simulink model "Detailed_PMSG_one_machine"  (Simulink 8.6)
settings: Solver=VariableStepAuto  StartTime=0.0  StopTime=30  FixedStep=Ts  MaxStep=Ts  RelTol=1e-3
PreLoadFcn:
  | Ts=5e-6;
InitFcn:
  | Ts=5e-6;
values from neighbouring files (symbols this model uses):
  A = c1*((c2/li-c3*u-c4)*exp(-c5/li))+c6*i    [Cpmax.m]    (also in deloaded_operation_with_pitch_angle.m = powercoefficient(tipmax,u))
undefined symbols (not defined in the file or in its folder): DiscIntNeverNeededParam, level
libraries: powerlib_extras x37, powerlib x21, simulink_extras x4, simulink x4, re_lib x1, sps_avr x1, powerlib_meascontrol x1
(part 2 of 2)

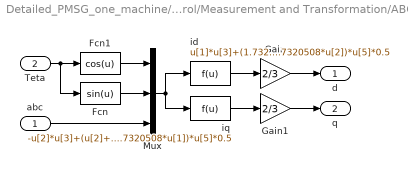
== system Detailed_PMSG_one_machine/PMSG Wind Turbine/Control/Measurement and Transformation/ABC to dq conversion ==
  abc : Inport
  Teta : Inport  Port=2
  Fcn : Fcn  Expr=sin(u)
  Fcn1 : Fcn  Expr=cos(u)
  Gain : Gain  Gain=2/3  SaturateOnIntegerOverflow=on  OutDataTypeStr=Inherit: Same as input  ParamDataTypeStr=Inherit: Same as input
  Gain1 : Gain  Gain=2/3  SaturateOnIntegerOverflow=on  OutDataTypeStr=Inherit: Same as input  ParamDataTypeStr=Inherit: Same as input
  Mux : Mux  Inputs=[1 1 3]
  id : Fcn  Expr=u[1]*u[3]+(1.7320508*u[2]-u[1])*u[4]*0.5+(-u[1]-1.7320508*u[2])*u[5]*0.5
  iq : Fcn  Expr=-u[2]*u[3]+(u[2]+1.7320508*u[1])*u[4]*0.5+(u[2]-1.7320508*u[1])*u[5]*0.5
  d : Outport  InitialOutput=0
  q : Outport  Port=2  InitialOutput=0
  wires:
  Fcn/1 -> Mux/2
  Fcn1/1 -> Mux/1
  Teta/1 -> Fcn1/1, Fcn/1
  Mux/1 -> iq/1, id/1
  abc/1 -> Mux/3
  iq/1 -> Gain1/1
  id/1 -> Gain/1
  Gain/1 -> d/1
  Gain1/1 -> q/1

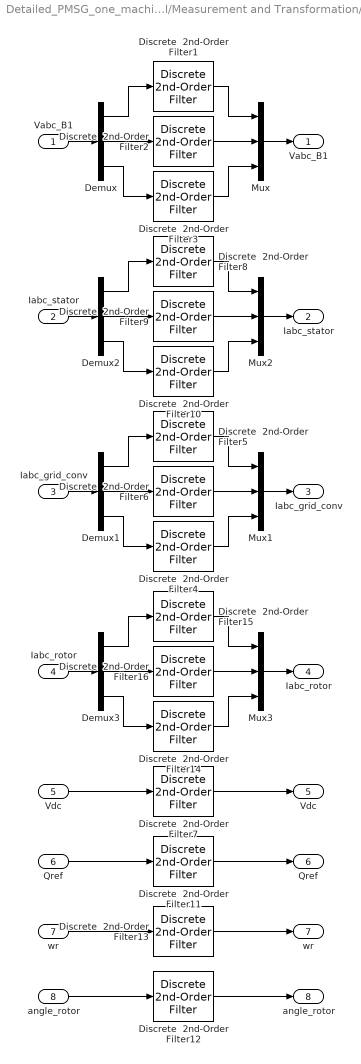
== system Detailed_PMSG_one_machine/PMSG Wind Turbine/Control/Measurement and Transformation/Filter ==
  Vabc_B1 : Inport
  Iabc_stator : Inport  Port=2
  Iabc_grid_conv : Inport  Port=3
  Iabc_rotor : Inport  Port=4
  Vdc : Inport  Port=5
  Qref : Inport  Port=6
  wr : Inport  Port=7
  angle_rotor : Inport  Port=8
  Demux{,1..3} (4 alike) : Demux  Outputs=3
  Discrete  2nd-Order Filter{1..6,8..16} (15 alike) : powerlib_extras/Discrete  Control Blocks/Discrete  2nd-Order Filter  FilterType=Lowpass  Fo=Freq  Zeta=Zeta1  Ts=Ts  Initialize=off  Vac_Init=[0.8 -25 60]  Vdc_Init=-0.4  PlotResponse=off  param1=[1 500 1]
  Discrete  2nd-Order Filter7 : powerlib_extras/Discrete  Control Blocks/Discrete  2nd-Order Filter  FilterType=Lowpass  Fo=Freq  Zeta=Zeta1  Ts=Ts  Initialize=on  Vac_Init=[0.8 -25 60]*0  Vdc_Init=Vdc_nom  PlotResponse=off  param1=[1 500 1]
  Mux{,1..3} (4 alike) : Mux  Inputs=3
  "Vabc_B1 " : Outport
  "Iabc_stator " : Outport  Port=2
  "Iabc_grid_conv " : Outport  Port=3
  "Iabc_rotor " : Outport  Port=4
  "Vdc " : Outport  Port=5
  "Qref " : Outport  Port=6
  "wr " : Outport  Port=7
  "angle_rotor " : Outport  Port=8
  wires:
  Discrete  2nd-Order Filter12/1 -> "angle_rotor "/1
  angle_rotor/1 -> Discrete  2nd-Order Filter12/1
  Discrete  2nd-Order Filter11/1 -> "Qref "/1
  Qref/1 -> Discrete  2nd-Order Filter11/1
  Mux3/1 -> "Iabc_rotor "/1
  Iabc_rotor/1 -> Demux3/1
  Discrete  2nd-Order Filter14/1 -> Mux3/3
  Discrete  2nd-Order Filter16/1 -> Mux3/2
  Discrete  2nd-Order Filter15/1 -> Mux3/1
  Demux3/3 -> Discrete  2nd-Order Filter14/1
  Demux3/2 -> Discrete  2nd-Order Filter16/1
  Demux3/1 -> Discrete  2nd-Order Filter15/1
  Discrete  2nd-Order Filter13/1 -> "wr "/1
  wr/1 -> Discrete  2nd-Order Filter13/1
  Mux2/1 -> "Iabc_stator "/1
  Iabc_stator/1 -> Demux2/1
  Discrete  2nd-Order Filter10/1 -> Mux2/3
  Discrete  2nd-Order Filter9/1 -> Mux2/2
  Discrete  2nd-Order Filter8/1 -> Mux2/1
  Demux2/3 -> Discrete  2nd-Order Filter10/1
  Demux2/2 -> Discrete  2nd-Order Filter9/1
  Demux2/1 -> Discrete  2nd-Order Filter8/1
  Discrete  2nd-Order Filter7/1 -> "Vdc "/1
  Vdc/1 -> Discrete  2nd-Order Filter7/1
  Mux1/1 -> "Iabc_grid_conv "/1
  Iabc_grid_conv/1 -> Demux1/1
  Discrete  2nd-Order Filter4/1 -> Mux1/3
  Discrete  2nd-Order Filter6/1 -> Mux1/2
  Discrete  2nd-Order Filter5/1 -> Mux1/1
  Demux1/3 -> Discrete  2nd-Order Filter4/1
  Demux1/2 -> Discrete  2nd-Order Filter6/1
  Demux1/1 -> Discrete  2nd-Order Filter5/1
  Mux/1 -> "Vabc_B1 "/1
  Vabc_B1/1 -> Demux/1
  Discrete  2nd-Order Filter3/1 -> Mux/3
  Discrete  2nd-Order Filter2/1 -> Mux/2
  Discrete  2nd-Order Filter1/1 -> Mux/1
  Demux/3 -> Discrete  2nd-Order Filter3/1
  Demux/2 -> Discrete  2nd-Order Filter2/1
  Demux/1 -> Discrete  2nd-Order Filter1/1

== system Detailed_PMSG_one_machine/PMSG Wind Turbine/Control/Rotor-side Controls/dq to ABC  conversion  ==
  dq : Inport
  Teta : Inport  Port=2
  Fcn : Fcn  Expr=sin(u)
  Fcn1 : Fcn  Expr=cos(u)
  Mux : Mux  Inputs=[1 1 2]
  Mux1 : Mux  Inputs=3
  a : Fcn  Expr=u(1)*u(3)-u(2)*u(4)
  b : Fcn  Expr=(u(1)*(-0.5)+u(2)*(0.8660254))*u(3)-(u(2)*(-0.5)-u(1)*(0.8660254))*u(4)
  c : Fcn  Expr=(u(1)*(-0.5)-u(2)*(0.8660254))*u(3)-(u(2)*(-0.5)+u(1)*(0.8660254))*u(4)
  ABC : Outport
  wires:
  Fcn/1 -> Mux/2
  Fcn1/1 -> Mux/1
  Teta/1 -> Fcn1/1, Fcn/1
  Mux/1 -> a/1, b/1, c/1
  dq/1 -> Mux/3
  b/1 -> Mux1/2
  a/1 -> Mux1/1
  Mux1/1 -> ABC/1
  c/1 -> Mux1/3

== matlab function PMSG Wind Turbine/MPPT/MATLAB Function ==
  data: u input double; tip output double; Cp output double
function [tip,Cp]= fcn(u)

c1 = 0.5176;
c2 = 116;
c3 = 0.4;
c4 = 5;
c5 = 21;
c6 = 0.0068;
B=0;
for i = 0.1:0.1:15
    
li = 1/((1/(i+0.08*u))-(0.035/(u^3+1)));
A = c1*((c2/li-c3*u-c4)*exp(-c5/li))+c6*i ;%#codegen

    if A < B
    lopt = i;
    break
    else 
    B = A;
    end
end
tip = i;
Cp = c1*((c2/li-c3*u-c4)*exp(-c5/li))+c6*i;
end
